simulink model "afmotor_v2"  (Simulink 8.0)
settings: Solver=FixedStepDiscrete  SolverMode=SingleTasking  StartTime=0.0  StopTime=10.0  RelTol=1e-3
settings Model: Creator=aapte  LastModifiedBy=gcampa  ExtModeTrigDuration=2
settings OptimizationCC: ExpressionDepthLimit=128  OptimizeModelRefInitCode=on  LifeSpan=1
settings DebuggingCC: SolverPrmCheckMsg=none  StrictBusMsg=Warning
settings HardwareCC: ProdBitPerInt=16  ProdBitPerPointer=8  ProdIntDivRoundTo=Zero  ProdEndianess=LittleEndian  ProdWordSize=8  ProdHWDeviceType=Atmel->AVR
settings RTWCC: SystemTargetFile=realtime.tlc  GenerateMakefile=off  TemplateMakefile=realtime.tmf  PostCodeGenCommand=setArduinoDefn(buildInfo)  Description=Run on Target Hardware  RTWVerbose=off  ProcessScript=realtime_make_rtw_hook  CustomSource=Wire.cpp twi.c Adafruit_PWMServoDriver.cpp  CustomLibrary=Adafruit_MotorShield.cpp
settings CodeAppCC: CustomSymbolStrType=$N$R$M_T
settings STFCustomTargetCC: TargetLibSuffix=.a  CodeReplacementLibrary=ANSI_C  GenerateSampleERTMain=on  ERTCustomFileBanners=on  SupportNonInlinedSFcns=off  SupportVariableSizeSignals=on  GRTInterface=off  SystemTargetFile=realtime.tlc
settings ERTTargetCC: CodeReplacementLibrary=ANSI_C  MultiwordLength=2048  GenerateSampleERTMain=on  ParMdlRefBuildCompliant=off  CompOptLevelCompliant=off  ConcurrentExecutionCompliant=off  CombineOutputUpdateFcns=off  ERTFirstTimeCompliant=off  SupportContinuousTime=on  SupportVariableSizeSignals=on  ModelStepFunctionPrototypeControlCompliant=off  CPPClassGenCompliant=off  ExtModeTransport=3  ExtModeMexFile=ext_serial_win32_comm  ExtModeMexArgs=0 1 9600  InlinedParameterPlacement=NonHierarchical  ERTSrcFileBannerTemplate=realtime_code_template.cgt  ERTHdrFileBannerTemplate=realtime_code_template.cgt  ERTDataSrcFileTemplate=realtime_code_template.cgt  ERTDataHdrFileTemplate=realtime_code_template.cgt  ERTCustomFileTemplate=realtime_file_process.tlc  ConvertIfToSwitch=off  SuppressUnreachableDefaultCases=off
settings SettingsController: Description=Run on Hardware Dialog  TargetExtensionPlatform=Arduino Uno
settings MATStruct: Set_host_COM_port=[1.0]  COM_port_number=4  COM_port_baud_rate=115200  Enable_overrun_detection=[0.0]  Digital_output_to_set_on_overrun=13  Analog_input_reference_voltage=[0.0]  Serial0_baud_rate=9600

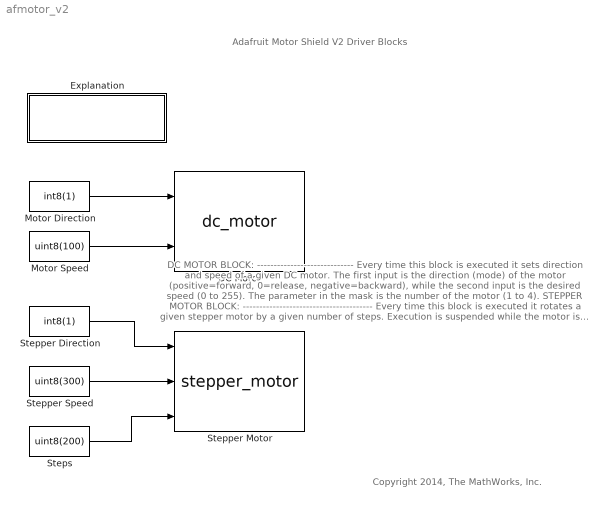
== system afmotor_v2 ==
  note: Copyright 2014, The MathWorks, Inc.
  note: DC MOTOR BLOCK:
      | -----------------------------
      | Every time this block is executed it sets direction and speed of a given DC motor.
      |
      | The first input is the direction (mode) of the motor (positive=forward, 0=release,
      | negative=backward), while the second input is the desired speed (0 to 255).
      | The parameter in the mask is the number of the motor (1 to 4).
      |
      |
      | STEPPER MOTOR BLOCK:
      | ---------------------------------------
      | Every time this block is executed it rotates a given stepper motor by a given
      | number of steps. Execution is suspended while the motor is running and is
      | resumed when the motor completes its rotation.
      |
      | The first input is the direction (mode) of the motor (positive=forward,
      | 0=release, negative=backward), the second input is the desired speed (0 to 255),
      | and the third is the number of desired steps (0 to 255). The first parameter in the
      | mask is the number of the stepper motor (1 or 2). The second parameter is the
      | motion style (single, double, interleave, microstep).
      |
      |
      | SEE ALSO:
      | ----------------
      | See AFMotorV2.pdf file for instructions on how to set up the blocks before use.
      | Also note that many of the block parameters are the same as the ones used in
      | the MATLAB Support Package for Arduino, so you might also have a look at that
      | package for additional explanations:
      | http://www.mathworks.com/matlabcentral/fileexchange/32374
  note: Adafruit Motor Shield V2 Driver Blocks
  DC Motor : S-Function  InitFcn=try, set_param(gcb,'FunctionName','dc_motor'), end  FunctionName=dc_motor  Parameters=uint8(1)  SFunctionModules=dc_motor_wrapper  WizardData=DataTag0  EnableBusSupport=off  mask(S-Function Builder){}
      mask help: Simulink:masks:SFunctionBuilder_MD
      mask init:
      | val = [[.9  0.75 0.75 1 1 .9 .9 1]',[1 1 0.75 0.75 .9 .9 1 .9]'];try , sys = get_param(gcb,'SfunBuilderFcnName');if isempty(sys), sys = get_param(gcb,'FunctionName'); end,catch, sys = get_param(gcb,'FunctionName'); end
      settings: PreSaveFcn=try, set_param(gcb,'FunctionName','dc_motor'), end  OpenFcn=sfunctionwizard(gcbh)
      settings: CopyFcn=|
      | set_param(gcbh,'LinkStatus','none')
      | setupMotorShieldv2(gcs)
      mask Display: plot(val(:,1),val(:,2)),disp(sys), port_label('input',1,'dir'), port_label('input',2,'spd')
  Explanation : Subsystem
      mask Display: disp('Double click \nfor setup explanation')
  Motor Direction : Constant  Value=int8(1)
  Motor Speed : Constant  Value=uint8(100)
  Stepper Direction : Constant  Value=int8(1)
  Stepper Motor : S-Function  InitFcn=try, set_param(gcb,'FunctionName','stepper_motor'), end  FunctionName=stepper_motor  Parameters=uint8(2),uint8(2)  SFunctionModules=stepper_motor_wrapper  WizardData=DataTag1  EnableBusSupport=off  mask(S-Function Builder){}
      mask help: Simulink:masks:SFunctionBuilder_MD
      mask init: same as afmotor_v2/DC Motor
      settings: PreSaveFcn=try, set_param(gcb,'FunctionName','stepper_motor'), end  OpenFcn=sfunctionwizard(gcbh)
      settings: CopyFcn=|
      | set_param(gcbh,'LinkStatus','none')
      | setupMotorShieldv2(gcs)
      mask Display: plot(val(:,1),val(:,2)),disp(sys), port_label('input',1,'dir'), port_label('input',2,'spd'), port_label('input',3,'stp')
  Stepper Speed : Constant  Value=uint8(300)
  Steps : Constant  Value=uint8(200)
  wires:
  Stepper Direction/1 -> Stepper Motor/1
  Stepper Speed/1 -> Stepper Motor/2
  Steps/1 -> Stepper Motor/3
  Motor Direction/1 -> DC Motor/1
  Motor Speed/1 -> DC Motor/2

== system afmotor_v2/Explanation ==
  note: GENERAL EXPLANATION:
      | --------------------------------------
      |
      | This model contains DC and Stepper Motor drivers for use with the (Arduino)
      | Adafruit Motor Shield Version 2 (http://www.adafruit.com/products/1438).
      |
      | Instructions below are also written in a better format in the AFMotorV2.pdf file.
      |
      |
      | RUNNING THE MODEL ON THE BOARD:
      | ----------------------------------------------------------
      |
      | To run the model on an arduino board you should:
      |
      | 1) run "SupportPackageInstaller" from the MATLAB command line and install the simulink
      | support package for arduino.
      |
      | 2) Make sure that the following files are in the current folder, (and that the folder
      | name does not contain any spaces):
      | afmotor_v2.mdl, setArduinoDefn.m, AFMotorV2Setup.m, renc2cpp.m, Wire.cpp,
      | Wire.h, twi.c, 	twi.h, Adafruit_MotorShield.cpp, Adafruit_MotorShield.h,
      | Adafruit_PWMServoDriver.cpp, Adafruit_PWMServoDriver.h
      | Note that the first 4 files are in the motorshields.zip file, Wire.* and twi.* are part of the
      | arduino IDE installation (e.g. C:\MATLAB\arduino-1.0.5), anf the last 4 files are part
      | of the AF Motor V2 Library.
      |
      | 3) Get rid of the redirection to the “utility” folder in line #22 of Adafruit_MotorShield.h
      | After the editing line #22 should be:
      | #include "Adafruit_PWMServoDriver.h"
      |
      | 4) Double-click on both the dc_motor and stepper motor blocks to open the S-Function interface,
      | then click on the Build button in right top corner to build the S-Functions. Then run the following
      | commands at the MATLAB command prompt:
      | >> renc2cpp('dc_motor');
      | >> renc2cpp('stepper_motor');
      |
      | 5) Click on “Tools > Run on Target Hardware > Prepare to run” (or, if you don’t see the
      | “Prepare to run” option click on “Tools > Run on Target Hardware > Options …”), and
      | make sure that the right board (e.g. Arduino Uno) and the right serial ports are selected.
      | Then click OK to save the settings.
      |
      | 6) Run the following command at the MATLAB command prompt:
      | >> AFMotorV2Setup('afmotor_v2');
      |
      | 7) Save the model and simulate it to check that there are no errors.
      | (The model should not do anything in simulation).
      |
      | 8) Make sure the Arduino is connected to the right serial port, that a DC motor
      | is connected to port 1 and a Stepper motor is connected to port 3 and 4, and
      | that no other program is using the serial port. (the best way to make sure
      | everything is good on the Arduino side is to test the motors with a small
      | example sketch like the one provided on the Adafruit site)
      |
      | 9) Click Tools > Run on Target Hardware > Run.
      | If everything goes well you should see both DC and Stepper motor running now.
      |
      | USING THE BLOCKS:
      | -------------------------------
      |
      | Note that every time you change a parameter in either the dc_motor or stepper_motor
      | blocks you will need to rebuild the S-Function and re-issue the respective ren2cpp call (step 4).
      | Also, if you change board or serial port, you’ll need to redo steps 5 and 6 above.
      |
      | If you create a new model and drag and drop either the dc_motor or stepper_motor blocks
      | you will need to redo steps 7 to 10 above, where in step 9 “afmotor_v2” must be replaced
      | with the name of the new model.
